simulink model "problema2"  (R2016a)
settings: Solver=FixedStepAuto  StartTime=0.0  StopTime=10.0  FixedStep=0.001  RelTol=1e-3
settings Model: Creator=usuario18  LastModifiedBy=usuario18

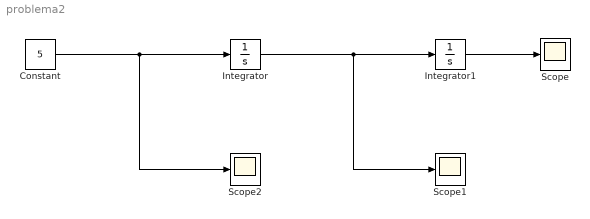
== system problema2 ==
  Constant : Constant  Value=5
  Integrator : Integrator
  Integrator1 : Integrator
  Scope : Scope
  Scope1 : Scope
  Scope2 : Scope
  wires:
  Constant/1 -> Integrator/1, Scope2/1
  Integrator/1 -> Scope1/1, Integrator1/1
  Integrator1/1 -> Scope/1
